simulink model "live"  (R2014a)
settings: Solver=FixedStepDiscrete  StartTime=0.0  StopTime=Inf  RelTol=1e-3
undefined symbols (not defined in the file): DiscIntNeverNeededParam
libraries: simulink x1
settings Model: Creator=eruffaldi  LastModifiedBy=eruffaldi

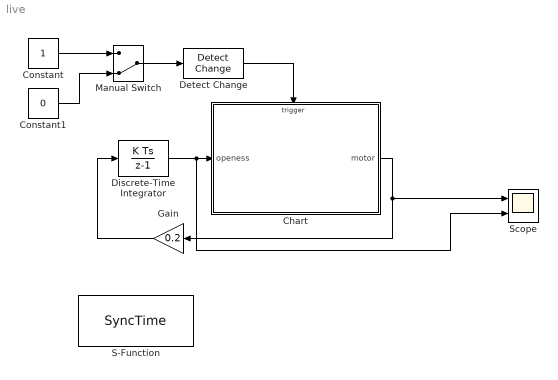
== system live ==
  Chart : Stateflow chart  TreatAsAtomicUnit=on
  Constant : Constant
  Constant1 : Constant  Value=0
  Detect Change : simulink/Logic and Bit Operations/Detect Change  vinit=0  InputProcessing=Inherited  OutDataTypeStr=boolean
  Discrete-Time Integrator : DiscreteIntegrator  LimitOutput=on  UpperSaturationLimit=1  LowerSaturationLimit=0  ICPrevOutput=DiscIntNeverNeededParam  ICPrevScaledInput=DiscIntNeverNeededParam
  Gain : Gain  Gain=0.2
  Manual Switch : ManualSwitch  CurrentSetting=0
  S-Function : S-Function  Priority=1024  FunctionName=SyncTime  Parameters=dt  EnableBusSupport=off  mask{dt=1/30}
      mask prompts: dt "Period (s) or 0 for sleepless"
      mask Display:
      | port_label('output',1,'Unix Epoch s');
      | port_label('output',2,'Slept s');
  Scope : Scope  NumInputPorts=2
      settings: YMin=1~1  YMax=1~1
  wires:
  Detect Change/1 -> Chart/Trigger
  Manual Switch/1 -> Detect Change/1
  Constant/1 -> Manual Switch/1
  Constant1/1 -> Manual Switch/2
  Discrete-Time Integrator/1 -> Scope/2, Chart/1(openess)
  Chart/1(motor) -> Scope/1, Gain/1
  Gain/1 -> Discrete-Time Integrator/1

== stateflow chart live/Chart ==
  state Ch
    en:
    motor=-1;
    ex:
    motor=0;
  state A
  state ChPause
  state C
  state Ap
    en:
    motor=1
    ex:
    motor = 0
  state ?
  A -> Ch [order 1] : button
  Ch -> ChPause [order 2] : button
  ChPause -> Ch : button
  A -> Ch [order 2] : after(10,sec)
  Ap -> A [order 1] : [openess >= 1]
  Ch -> C [order 1] : [openess <= 0]
  (default) -> C
  C -> Ap : button
  Ap -> ? [order 2] : button
  ? -> Ap : button
  data: openess input double size=1; motor output double size=1
  events: button input EITHER_EDGE_EVENT
